simulink model "modem_8QAM_v2018b"  (R2018b)
settings: Solver=VariableStepAuto  StartTime=0.0  StopTime=tsym+(1/3000000)  RelTol=1e-3
libraries: simulink x6, dspsigops x2, dspsrcs4 x1
settings Model: SimulationMode=accelerator  Creator=mparada  LastModifiedBy=brunocasu
settings SFSimCC: SimUseLocalCustomCode=off
settings RTWCC: RTWUseLocalCustomCode=off

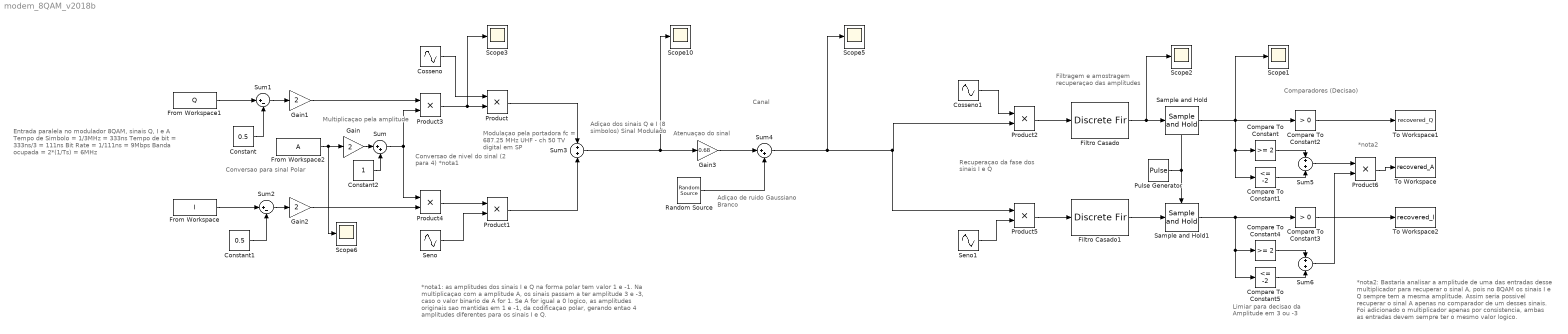
== system modem_8QAM_v2018b ==
  note: Conversao para
      | sinal Polar
  note: Modulaçao pela
      | portadora
      | fc = 687.25 MHz
      | UHF - ch 50 TV digital em SP
  note: Adiçao dos sinais
      | Q e I (8 simbolos)
      | Sinal Modulado
  note: Multiplicaçao
      | pela amplitude
  note: Conversao de nivel
      | do sinal (2 para 4)
      | *nota1
  note: Recuperaçao da fase
      | dos sinais I e Q
  note: Filtragem e amostragem
      | recuperaçao das amplitudes
  note: Comparadores
      | (Decisao)
  note: *nota2
  note: *nota2:
      | Bastaria analisar a amplitude de uma das entradas
      | desse multiplicador para recuperar o sinal A, pois no
      | 8QAM os sinais I e Q sempre tem a mesma amplitude.
      | Assim seria possivel recuperar o sinal A apenas no
      | comparador de um desses sinais.
      | Foi adicionado o multiplicador apenas por consistencia,
      | ambas as entradas devem sempre ter o mesmo valor logico.
  note: Adiçao de ruido
      | Gaussiano Branco
  note: Canal
  note: *nota1:
      | as amplitudes dos sinais I e Q na forma polar tem
      | valor 1 e -1.
      | Na multiplicaçao com a amplitude A, os sinais passam
      | a ter amplitude 3 e -3, caso o valor binario de A for 1.
      | Se A for igual a 0 logico, as amplitudes originais sao mantidas
      | em 1 e -1, da codificaçao polar, gerando entao 4 amplitudes diferentes
      | para os sinais I e Q.
  note: Entrada paralela no modulador 8QAM, sinais Q, I e A
      |
      | Tempo de Simbolo = 1/3MHz = 333ns
      | Tempo de bit = 333ns/3 = 111ns
      | Bit Rate = 1/111ns = 9Mbps
      | Banda ocupada = 2*(1/Ts) = 6MHz
  note: Limiar para decisao da
      | Amplitude em 3 ou -3
  note: Atenuaçao do sinal
  Compare To Constant : simulink/Logic and Bit Operations/Compare To Constant  relop=>=  const=2  OutDataTypeStr=boolean
  Compare To Constant1 : simulink/Logic and Bit Operations/Compare To Constant  relop=<=  const=-2  OutDataTypeStr=boolean
  Compare To Constant2 : simulink/Logic and Bit Operations/Compare To Constant  relop=>  const=0  OutDataTypeStr=boolean
  Compare To Constant3 : simulink/Logic and Bit Operations/Compare To Constant  relop=>  const=0  OutDataTypeStr=boolean
  Compare To Constant4 : simulink/Logic and Bit Operations/Compare To Constant  relop=>=  const=2  OutDataTypeStr=boolean
  Compare To Constant5 : simulink/Logic and Bit Operations/Compare To Constant  relop=<=  const=-2  OutDataTypeStr=boolean
  Constant : Constant  Value=0.5
  Constant1 : Constant  Value=0.5
  Constant2 : Constant
  Cosseno : Sin  Frequency=2*pi*687250000  Phase=pi/2  SampleTime=1/6872500000
  Cosseno1 : Sin  Frequency=2*pi*687250000  Phase=pi/2  SampleTime=1/6872500000
  Filtro Casado : DiscreteFir  Coefficients=ones(1,2290)/1145  SampleTime=1/6872500000
  Filtro Casado1 : DiscreteFir  Coefficients=ones(1,2290)/1145  SampleTime=1/6872500000
  From Workspace : FromWorkspace  VariableName=I  SampleTime=1/3000000  Interpolate=off  OutputAfterFinalValue=Setting to zero
  From Workspace1 : FromWorkspace  VariableName=Q  SampleTime=1/3000000  Interpolate=off  OutputAfterFinalValue=Setting to zero
  From Workspace2 : FromWorkspace  VariableName=A  SampleTime=1/3000000  Interpolate=off  OutputAfterFinalValue=Setting to zero
  Gain : Gain  Gain=2
  Gain1 : Gain  Gain=2
  Gain2 : Gain  Gain=2
  Gain3 : Gain  Gain=0.68
  Product{,1..6} (7 alike) : Product
  Pulse Generator : DiscretePulseGenerator  PulseType=Time based  Period=1/3000000  PulseWidth=0.00001  PhaseDelay=1/3000000
  Random Source : dspsrcs4/Random Source  SrcType=Gaussian  NormMethod=Ziggurat  CltLength=12  MinVal=0  MaxVal=1  MeanVal=0  VarVal=2  RepMode=Not repeatable  rawSeed=1  IsInherit=off  SampMode=Discrete  SampTime=1/300000000  SampFrame=1  DataType=Double  OutComplex=Real  OutputFrames=off
  Sample and Hold : dspsigops/Sample and Hold  trig=Rising edge  initCond=0  latchinput=off
  Sample and Hold1 : dspsigops/Sample and Hold  trig=Rising edge  initCond=0  latchinput=off
  Scope{1..3,5..6,10} (6 alike) : Scope
  Seno : Sin  Frequency=2*pi*687250000  SampleTime=1/6872500000
  Seno1 : Sin  Frequency=2*pi*687250000  SampleTime=1/6872500000
  Sum : Sum  Inputs=|++
  Sum1 : Sum  Inputs=|+-
  Sum2 : Sum  Inputs=|+-
  Sum3 : Sum  Inputs=+|+
  Sum4 : Sum  Inputs=|++
  Sum5 : Sum  Inputs=+|+
  Sum6 : Sum  Inputs=+|+
  To Workspace : ToWorkspace  VariableName=recovered_A  SaveFormat=Structure With Time  SampleTime=1/3000000
  To Workspace1 : ToWorkspace  VariableName=recovered_Q  SaveFormat=Structure With Time  SampleTime=1/3000000
  To Workspace2 : ToWorkspace  VariableName=recovered_I  SaveFormat=Structure With Time  SampleTime=1/3000000
  wires:
  Constant/1 -> Sum1/2
  Constant1/1 -> Sum2/2
  From Workspace/1 -> Sum2/1
  From Workspace1/1 -> Sum1/1
  Sum2/1 -> Gain2/1
  Sum1/1 -> Gain1/1
  Gain/1 -> Sum/1
  Constant2/1 -> Sum/2
  From Workspace2/1 -> Scope6/1, Gain/1
  Seno/1 -> Product1/2
  Product/1 -> Sum3/1
  Sum3/1 -> Scope10/1, Gain3/1
  Gain1/1 -> Product3/1
  Sum/1 -> Product4/1, Product3/2
  Gain2/1 -> Product4/2
  Product3/1 -> Scope3/1, Product/2
  Product4/1 -> Product1/1
  Product1/1 -> Sum3/2
  Random Source/1 -> Sum4/2
  Cosseno1/1 -> Product2/1
  Seno1/1 -> Product5/2
  Compare To Constant/1 -> Sum5/1
  Compare To Constant1/1 -> Sum5/2
  Pulse Generator/1 -> Sample and Hold1/Trigger, Sample and Hold/Trigger
  Sample and Hold/1 -> Scope1/1, Compare To Constant2/1, Compare To Constant1/1, Compare To Constant/1
  Compare To Constant2/1 -> To Workspace1/1
  Compare To Constant3/1 -> To Workspace2/1
  Product6/1 -> To Workspace/1
  Sample and Hold1/1 -> Compare To Constant5/1, Compare To Constant4/1, Compare To Constant3/1
  Compare To Constant5/1 -> Sum6/2
  Compare To Constant4/1 -> Sum6/1
  Sum6/1 -> Product6/2
  Sum5/1 -> Product6/1
  Gain3/1 -> Sum4/1
  Sum4/1 -> Scope5/1, Product5/1, Product2/2
  Product2/1 -> Filtro Casado/1
  Product5/1 -> Filtro Casado1/1
  Filtro Casado/1 -> Scope2/1, Sample and Hold/1
  Filtro Casado1/1 -> Sample and Hold1/1
  Cosseno/1 -> Product/1
